simulink model "sampleModel1532"  (R2023a)
settings: Solver=VariableStepAuto  StartTime=0.0  StopTime=10.0  RelTol=1e-3
libraries: hdlsllib x4, simulink x1
settings Model: Creator=user1  LastModifiedBy=user1

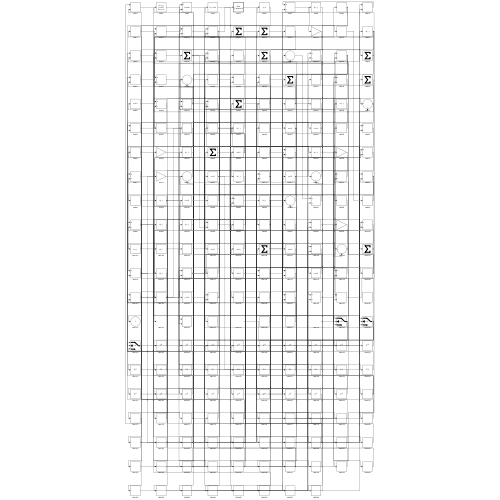
[thumbnail: Simulink's stored preview of the top-level diagram]
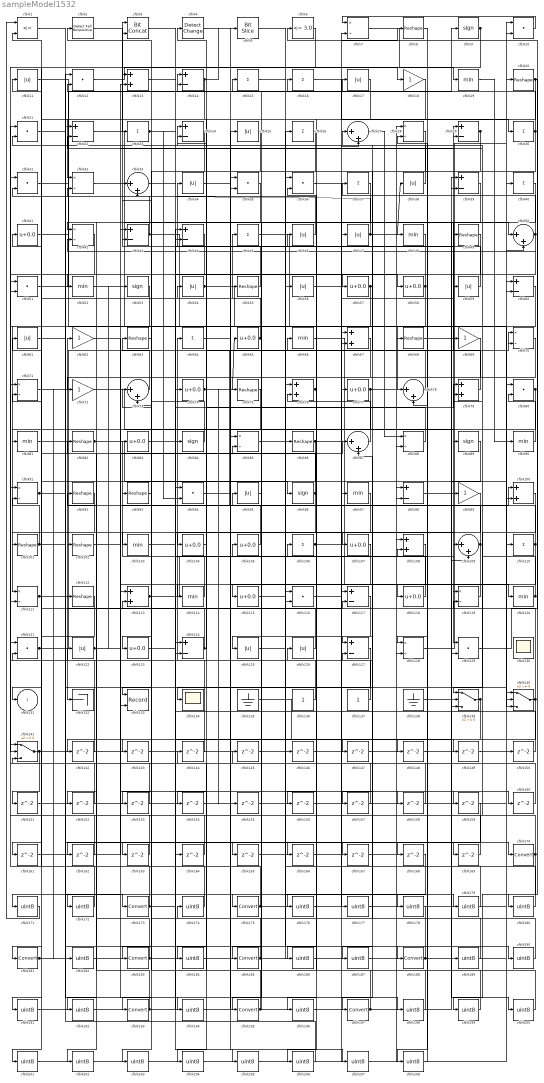
== system sampleModel1532 ==
  cfblk1 : RelationalOperator  Operator=<=  OutDataTypeStr=boolean  InputSameDT=off
  cfblk{10,12,21,31,35..36,51,80,94,116,121,129} (12 alike) : DotProduct  OutDataTypeStr=Inherit: Inherit via internal rule
  cfblk{13,67,76,79,100,108,113} (7 alike) : Sum
  cfblk{8,20,49,55,63,68,75,82,86,92..93,101..102,112} (14 alike) : Reshape
  cfblk{19,48,52,66,81,90,97,103,114,120} (10 alike) : MinMax
  cfblk{41,57..58,65,74,77,83,104..105,107,115,118,123} (13 alike) : Bias  Bias=0.0  SaturateOnIntegerOverflow=off
  cfblk{15..16,23,26,30,37,40,45,64,106,110} (11 alike) : Sum  Inputs=+
  cfblk{27,33,50,73,78,87,109} (7 alike) : Sum  Inputs=|++
  cfblk{11,17,25,34,38,46..47,54,56,59,61,95,122,125..126} (15 alike) : Abs  SaturateOnIntegerOverflow=off
  cfblk{7,28,32,42,70..71,85,88,91,111,119,128} (12 alike) : Product  Inputs=*/  RndMeth=Zero  SaturateOnIntegerOverflow=on
  cfblk{14,22,24,29,39,43..44,60,98,117,124,127} (12 alike) : Sum  Inputs=+-
  cfblk130 : Scope
      settings: Floating=on
  cfblk132 : Terminator
  cfblk133 : Record  FileSettingsInternal="{\"entries\":[{\"content\":{\"excelSettings\":{\"content\":{},\"type\":\"Streamout.ExcelSettings\"}},\"type\":\"Streamout.FileSettingStorage\",\"uuid\":\"\"}],\"packageUris\":[\"http:\\/\\/schema.mathworks.com\\/mf0\\/streamout_blocks\\/R2020a\"],\"version\":\"1.0\"}"  Layout=[1 1]  SignalsInternal="{\"entries\":[{\"content\":{\"signals\":[{\"content\":{\"blockPath\":[],\"dimensions\":[1],\"domain\":\"\",\"lineColor\":\"#a2142f\",\"plots\":[1],\"port\":1,\"signalID\":1555,\"signalName\":\"XY Graph:1\"},\"type\":\"RecordBlkView.Signal\",\"uuid\":\"\"},{\"content\":{\"blockPath\":[],\"dimensions\":[1],\"domain\":\"\",\"lineColor\":\"#139fff\",\"plots\":[1],\"port\":2,\"signalID\":1558,\"signalName\":\"XY Graph:2\"},\"type\":\"RecordBlkView.Signal\",\"uuid\":\"\"}]},\"type\":\"RecordBlkView.InputSignals\",\"uuid\":\"\"}],\"packageUris\":[\"http:\\/\\/schema.mathworks.com\\/mf0\\/streamout_blocks\\/R2020a\"],\"version\":\"1.0\"}"  VisualizationBindings="{\"xyplotplugin\":{\"info\":[{\"series\":[{\"bindingParametersList\":[{\"parameter\":\"X-Axis\",\"signalID\":1555,\"signalName\":\"XY Graph:1\"},{\"parameter\":\"Y-Axis\",\"signalID\":1558,\"signalName\":\"XY Graph:2\"}],\"seriesID\":30679}],\"subplotID\":1}]}}"  CompatibilityTag=XY  st=-1
  cfblk134 : Scope
  cfblk135 : Ground
  cfblk136 : Constant  SampleTime=-1
  cfblk137 : Constant  SampleTime=-1
  cfblk138 : Ground
  cfblk139 : Switch  SaturateOnIntegerOverflow=off  InputSameDT=off
  cfblk140 : Switch  SaturateOnIntegerOverflow=off  InputSameDT=off
  cfblk141 : Switch  SaturateOnIntegerOverflow=off  InputSameDT=off
  cfblk{142..169} (28 alike) : Delay  SampleTime=1
  cfblk{170,173,175,181,183,185,188,193,195,197} (10 alike) : DataTypeConversion  SaturateOnIntegerOverflow=off  RndMeth=Floor
  cfblk{171..172,174,176..180,182,184,186..187,189..192,194,196,198..208} (29 alike) : DataTypeConversion  OutDataTypeStr=uint8  SaturateOnIntegerOverflow=off  RndMeth=Floor
  cfblk{18,62,69,72,99} (5 alike) : Gain
  cfblk2 : hdlsllib/Logic and Bit Operations/Detect Fall Nonpositive  vinit=0  OutDataTypeStr=boolean
  cfblk3 : hdlsllib/Logic and Bit Operations/Bit Concat  numInputs=2
  cfblk4 : simulink/Logic and Bit Operations/Detect Change  vinit=0  OutDataTypeStr=boolean
      settings: LibrarySourceBlock=|
      | hdlsllib/Logic and Bit
      | Operations/Detect
      | Change
  cfblk5 : hdlsllib/Logic and Bit Operations/Bit Slice  lidx=7  ridx=0
  cfblk{9,53,84,89,96} (5 alike) : Signum
  cfblk6 : hdlsllib/Logic and Bit Operations/Compare To Constant  relop=<=  const=3.0  OutDataTypeStr=boolean
  cfblk131 : Outport  VectorParamsAs1DForOutWhenUnconnected=off
  wires:
  cfblk1/1 -> cfblk170/1
  cfblk19/1 -> cfblk90/1
  cfblk41/1 -> cfblk17/1
  cfblk27/1 -> cfblk88/1
  cfblk92/1 -> cfblk132/1
  cfblk71/1 -> cfblk62/1
  cfblk110/1 -> cfblk125/1, cfblk14/1
  cfblk73/1 -> cfblk63/1
  cfblk31/1 -> cfblk16/1
  cfblk129/1 -> cfblk6/1
  cfblk55/1 -> cfblk34/1
  cfblk58/1 -> cfblk111/1, cfblk52/1
  cfblk7/1 -> cfblk19/1
  cfblk105/1 -> cfblk66/1
  cfblk136/1 -> cfblk64/1
  cfblk16/1 -> cfblk30/1
  cfblk45/1 -> cfblk78/1
  cfblk11/1 -> cfblk68/1
  cfblk29/1 -> cfblk127/1, cfblk157/1, cfblk196/1
  cfblk124/1 -> cfblk11/1, cfblk14/2
  cfblk82/1 -> cfblk96/1, cfblk29/2
  cfblk120/1 -> cfblk24/1, cfblk22/2
  cfblk121/1 -> cfblk100/1, cfblk74/1
  cfblk14/1 -> cfblk5/1, cfblk32/1
  cfblk65/1 -> cfblk45/1, cfblk41/1
  cfblk81/1 -> cfblk25/1
  cfblk66/1 -> cfblk120/1
  cfblk141/1 -> cfblk35/2, cfblk151/1
  cfblk39/1 -> cfblk175/1
  cfblk33/1 -> cfblk107/1
  cfblk61/1 -> cfblk173/1
  cfblk22/1 -> cfblk110/1
  cfblk4/1 -> cfblk50/1
  cfblk111/1 -> cfblk29/1, cfblk72/1, cfblk182/1
  cfblk18/1 -> cfblk131/1
  cfblk78/1 -> cfblk24/2
  cfblk74/1 -> cfblk65/1, cfblk155/1
  cfblk59/1 -> cfblk3/1
  cfblk87/1 -> cfblk76/2
  cfblk108/1 -> cfblk197/1
  cfblk128/1 -> cfblk70/1
  cfblk26/1 -> cfblk183/1
  cfblk97/1 -> cfblk195/1
  cfblk47/1 -> cfblk38/1, cfblk33/2
  cfblk85/1 -> cfblk188/1
  cfblk57/1 -> cfblk104/1, cfblk167/1
  cfblk113/1 -> cfblk10/2, cfblk106/1
  cfblk6/1 -> cfblk51/2
  cfblk51/1 -> cfblk9/1
  cfblk79/1 -> cfblk27/1
  cfblk119/1 -> cfblk115/1
  cfblk140/1 -> cfblk73/2, cfblk148/1, cfblk149/1, cfblk176/1
  cfblk86/1 -> cfblk8/1, cfblk160/1, cfblk161/1, cfblk162/1
  cfblk13/1 -> cfblk84/1
  cfblk38/1 -> cfblk21/2
  cfblk43/1 -> cfblk140/1, cfblk32/2
  cfblk25/1 -> cfblk134/1
  cfblk49/1 -> cfblk123/1
  cfblk50/1 -> cfblk57/1, cfblk37/1, cfblk42/2
  cfblk69/1 -> cfblk112/1
  cfblk2/1 -> cfblk23/1
  cfblk89/1 -> cfblk102/1
  cfblk52/1 -> cfblk117/1
  cfblk76/1 -> cfblk46/1, cfblk166/1
  cfblk40/1 -> cfblk129/1
  cfblk103/1 -> cfblk49/1
  cfblk23/1 -> cfblk94/2, cfblk58/1, cfblk147/1
  cfblk48/1 -> cfblk181/1
  cfblk24/1 -> cfblk133/1
  cfblk60/1 -> cfblk185/1
  cfblk12/1 -> cfblk18/1
  cfblk114/1 -> cfblk83/1
  cfblk54/1 -> cfblk119/1, cfblk169/1
  cfblk101/1 -> cfblk91/2, cfblk139/3
  cfblk95/1 -> cfblk55/1
  cfblk139/1 -> cfblk152/1, cfblk153/1
  cfblk138/1 -> cfblk69/1
  cfblk72/1 -> cfblk89/1
  cfblk5/1 -> cfblk109/1
  cfblk126/1 -> cfblk54/1
  cfblk9/1 -> cfblk78/2, cfblk101/1
  cfblk84/1 -> cfblk2/1
  cfblk20/1 -> cfblk12/2, cfblk156/1, cfblk180/1
  cfblk90/1 -> cfblk80/2
  cfblk56/1 -> cfblk47/1
  cfblk125/1 -> cfblk56/1
  cfblk80/1 -> cfblk114/1, cfblk81/1
  cfblk116/1 -> cfblk77/1
  cfblk68/1 -> cfblk100/2
  cfblk15/1 -> cfblk140/2
  cfblk77/1 -> cfblk70/2, cfblk192/1
  cfblk10/1 -> cfblk7/1
  cfblk94/1 -> cfblk118/1
  cfblk83/1 -> cfblk79/1
  cfblk75/1 -> cfblk193/1
  cfblk46/1 -> cfblk31/2
  cfblk109/1 -> cfblk133/2, cfblk93/1
  cfblk8/1 -> cfblk128/1
  cfblk30/1 -> cfblk13/1, cfblk208/1
  cfblk32/1 -> cfblk109/2
  cfblk35/1 -> cfblk42/1
  cfblk53/1 -> cfblk141/2
  cfblk100/1 -> cfblk139/1
  cfblk118/1 -> cfblk43/2
  cfblk96/1 -> cfblk116/2, cfblk71/2
  cfblk137/1 -> cfblk92/1
  cfblk122/1 -> cfblk87/1, cfblk117/2, cfblk53/1
  cfblk88/1 -> cfblk4/1
  cfblk106/1 -> cfblk140/3, cfblk59/1
  cfblk63/1 -> cfblk103/1
  cfblk91/1 -> cfblk139/2, cfblk194/1
  cfblk42/1 -> cfblk111/2
  cfblk70/1 -> cfblk142/1
  cfblk142/1 -> cfblk91/1
  cfblk44/1 -> cfblk143/1
  cfblk143/1 -> cfblk116/1
  cfblk144/1 -> cfblk51/1
  cfblk145/1 -> cfblk129/2
  cfblk146/1 -> cfblk10/1
  cfblk148/1 -> cfblk80/1
  cfblk149/1 -> cfblk79/2
  cfblk150/1 -> cfblk94/1
  cfblk151/1 -> cfblk76/1
  cfblk152/1 -> cfblk31/1
  cfblk153/1 -> cfblk121/2
  cfblk17/1 -> cfblk154/1
  cfblk154/1 -> cfblk50/2
  cfblk157/1 -> cfblk71/1
  cfblk34/1 -> cfblk158/1
  cfblk158/1 -> cfblk35/1
  cfblk102/1 -> cfblk159/1
  cfblk160/1 -> cfblk141/1
  cfblk161/1 -> cfblk13/2
  cfblk162/1 -> cfblk22/1
  cfblk93/1 -> cfblk163/1
  cfblk163/1 -> cfblk43/1
  cfblk123/1 -> cfblk164/1
  cfblk164/1 -> cfblk21/1
  cfblk117/1 -> cfblk165/1
  cfblk165/1 -> cfblk27/2
  cfblk166/1 -> cfblk7/2
  cfblk167/1 -> cfblk88/2
  cfblk115/1 -> cfblk168/1
  cfblk169/1 -> cfblk113/1
  cfblk170/1 -> cfblk127/2, cfblk119/2, cfblk105/1, cfblk199/1
  cfblk168/1 -> cfblk171/1
  cfblk171/1 -> cfblk1/1
  cfblk159/1 -> cfblk172/1
  cfblk172/1 -> cfblk1/2
  cfblk173/1 -> cfblk44/2, cfblk121/1
  cfblk174/1 -> cfblk61/1
  cfblk175/1 -> cfblk150/1, cfblk73/1, cfblk141/3
  cfblk176/1 -> cfblk39/1
  cfblk156/1 -> cfblk177/1
  cfblk177/1 -> cfblk39/2
  cfblk36/1 -> cfblk178/1
  cfblk178/1 -> cfblk174/1
  cfblk155/1 -> cfblk179/1
  cfblk179/1 -> cfblk36/1
  cfblk180/1 -> cfblk36/2
  cfblk181/1 -> cfblk124/1, cfblk86/1
  cfblk182/1 -> cfblk48/1
  cfblk183/1 -> cfblk146/1, cfblk122/1
  cfblk104/1 -> cfblk184/1
  cfblk184/1 -> cfblk26/1
  cfblk185/1 -> cfblk145/1, cfblk113/2
  cfblk107/1 -> cfblk186/1
  cfblk186/1 -> cfblk60/1
  cfblk147/1 -> cfblk187/1
  cfblk187/1 -> cfblk60/2
  cfblk188/1 -> cfblk15/1, cfblk87/2, cfblk40/1
  cfblk135/1 -> cfblk189/1
  cfblk189/1 -> cfblk85/1
  cfblk21/1 -> cfblk190/1
  cfblk190/1 -> cfblk85/2
  cfblk99/1 -> cfblk191/1
  cfblk191/1 -> cfblk44/1
  cfblk192/1 -> cfblk99/1
  cfblk193/1 -> cfblk124/2, cfblk82/1
  cfblk194/1 -> cfblk75/1
  cfblk195/1 -> cfblk3/2, cfblk128/2, cfblk95/1
  cfblk196/1 -> cfblk97/1
  cfblk197/1 -> cfblk144/1, cfblk33/1
  cfblk62/1 -> cfblk198/1
  cfblk198/1 -> cfblk108/1
  cfblk199/1 -> cfblk108/2
  cfblk98/1 -> cfblk200/1
  cfblk200/1 -> cfblk126/1
  cfblk112/1 -> cfblk201/1
  cfblk201/1 -> cfblk98/1
  cfblk37/1 -> cfblk202/1
  cfblk202/1 -> cfblk98/2
  cfblk67/1 -> cfblk203/1
  cfblk203/1 -> cfblk20/1
  cfblk127/1 -> cfblk204/1
  cfblk204/1 -> cfblk67/1
  cfblk3/1 -> cfblk205/1
  cfblk205/1 -> cfblk67/2
  cfblk28/1 -> cfblk206/1
  cfblk206/1 -> cfblk12/1
  cfblk64/1 -> cfblk207/1
  cfblk207/1 -> cfblk28/1
  cfblk208/1 -> cfblk28/2
